simulink model "quatConversion_th"  (R2022a)
settings: Solver=VariableStepAuto  StartTime=0.0  StopTime=0  RelTol=1e-3
values from neighbouring files (symbols this model uses):
  eulAng = 2*(rand(3,1)-0.5)*90    [quatConversion_ts.m]
libraries: sharedtransform x2, eulAng2RotMat_ul x1, vectorNormalizer_ul x1, quat2EulerAng_ul x1, rotMat2Quat_ul x1
settings Model: Creator=mcobb  LastModifiedBy=lhill8
settings SolverCC: AlgebraicLoopSolver=TrustRegion
settings DebuggingCC: UnconnectedInputMsg=warning  UnconnectedOutputMsg=warning  UnconnectedLineMsg=warning  SFMachineParentedDataDiag=warning  ArithmeticOperatorsInVariantConditions=warning
settings SFSimCC: CustomCodeUndefinedFunction=UseInterfaceOnly

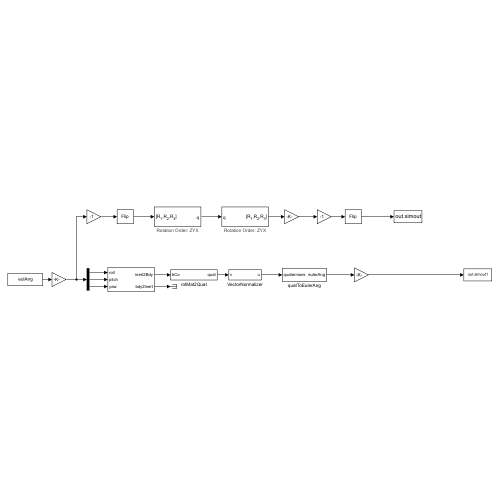
[thumbnail: Simulink's stored preview of the top-level diagram]
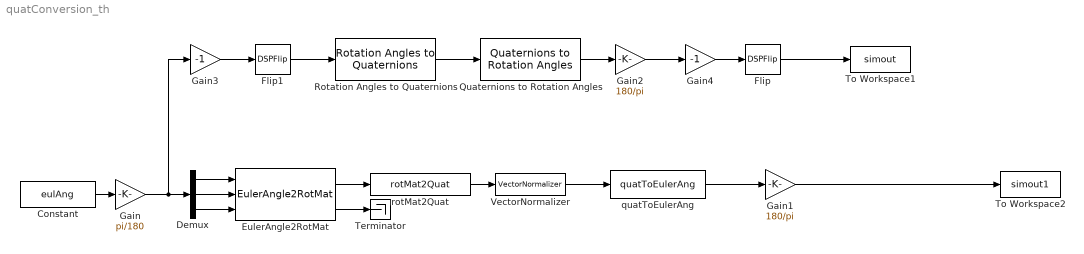
== system quatConversion_th ==
  Constant : Constant  Value=eulAng
  Demux : Demux  Outputs=3
  EulerAngle2RotMat : eulAng2RotMat_ul/EulerAngle2RotMat  SystemSampleTime=-1  VariantActivationTime=update diagram  Latency=0  AutoFrameSizeCalculation=off
  Flip : DSPFlip
  Flip1 : DSPFlip
  Gain : Gain  Gain=pi/180
  Gain1 : Gain  Gain=180/pi
  Gain2 : Gain  Gain=180/pi
  Gain3 : Gain  Gain=-1
  Gain4 : Gain  Gain=-1
  Quaternions to Rotation Angles : sharedtransform/Quaternions to Rotation Angles  rotationOrder=ZYX  aMode=aMode
      settings: SourceProductBaseCode=AE,PW,DR,MT,VE
  Rotation Angles to Quaternions : sharedtransform/Rotation Angles to Quaternions  rotationOrder=ZYX  aMode=aMode
      settings: SourceProductBaseCode=AE,PW,DR,MT,VE
  Terminator : Terminator
  To Workspace1 : ToWorkspace  VariableName=simout  SaveFormat=Timeseries  SampleTime=-1
  To Workspace2 : ToWorkspace  VariableName=simout1  SaveFormat=Timeseries  SampleTime=-1
  "VectorNormalizer " : vectorNormalizer_ul/VectorNormalizer   SystemSampleTime=-1  VariantActivationTime=update diagram  Latency=0  AutoFrameSizeCalculation=off
  quatToEulerAng : quat2EulerAng_ul/quatToEulerAng  SystemSampleTime=-1  VariantActivationTime=update diagram  Latency=0  AutoFrameSizeCalculation=off
  rotMat2Quat : rotMat2Quat_ul/rotMat2Quat  SystemSampleTime=-1  VariantActivationTime=update diagram  Latency=0  AutoFrameSizeCalculation=off
  wires:
  rotMat2Quat/1 -> "VectorNormalizer "/1
  EulerAngle2RotMat/1 -> rotMat2Quat/1
  EulerAngle2RotMat/2 -> Terminator/1
  Demux/2 -> EulerAngle2RotMat/2
  Demux/1 -> EulerAngle2RotMat/1
  Demux/3 -> EulerAngle2RotMat/3
  Constant/1 -> Gain/1
  "VectorNormalizer "/1 -> quatToEulerAng/1
  Gain/1 -> Gain3/1, Demux/1
  quatToEulerAng/1 -> Gain1/1
  Gain1/1 -> To Workspace2/1
  Quaternions to Rotation Angles/1 -> Gain2/1
  Gain2/1 -> Gain4/1
  Flip/1 -> To Workspace1/1
  Flip1/1 -> Rotation Angles to Quaternions/1
  Gain3/1 -> Flip1/1
  Rotation Angles to Quaternions/1 -> Quaternions to Rotation Angles/1
  Gain4/1 -> Flip/1
